simulink library "csu_esf_est_switch_frame_lib"  (R2015b)
settings: Solver=ode45  StartTime=0.0  StopTime=10.0  RelTol=1e-3
values from neighbouring files (symbols this model uses):
  esf_takeoff_accel_limit = 1.05    [csu_esf_est_switch_frame_init.m]
undefined symbols (not defined in the file or in its folder): ekf_covariance_init, kfl_accel_init, kfl_altitude_init, kfl_convergence_init, kfl_landed_init, kfl_quat_init, kfl_rate_init, kfl_state_init
libraries: simulink x2, util_info_lib x2, csu_egm_estimated_gravity_model_lib x2, util_fsw_frame_rotation_lib x2, util_common_lib x2
settings Model: Creator=escrane  LastModifiedBy=Mark Agbayani
settings DataIOCC: SaveFormat=Array
settings DebuggingCC: UnderspecifiedInitializationDetection=Classic  MergeDetectMultiDrivingBlocksExec=none  SolverPrmCheckMsg=warning  StateNameClashWarn=warning
settings HardwareCC: ProdBitPerPointer=32  ProdLargestAtomicFloat=None  ProdIntDivRoundTo=Undefined  ProdEndianess=Unspecified  ProdWordSize=32  ProdHWDeviceType=32-bit Generic
settings GRTTargetCC: GeneratePreprocessorConditionals=Disable all
settings ConfigComp: CovModelRefEnable=Off  CovSFcnEnable=off

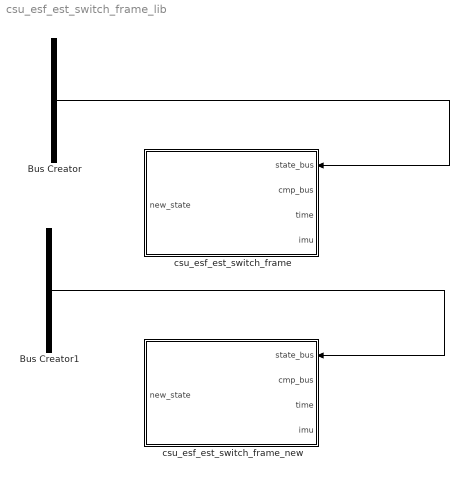
== system csu_esf_est_switch_frame_lib ==
  Bus Creator : BusCreator  Inputs=5
  Bus Creator1 : BusCreator  Inputs=6
  csu_esf_est_switch_frame : Subsystem
  csu_esf_est_switch_frame_new : Subsystem
  wires:
  Bus Creator/1 -> csu_esf_est_switch_frame/1(state_bus)
  ? -> Bus Creator/1  "x"
  ? -> Bus Creator/2  "accel"
  ? -> Bus Creator/3  "rate"
  ? -> Bus Creator/4  "q"
  ? -> Bus Creator/5  "P"
  Bus Creator1/1 -> csu_esf_est_switch_frame_new/1(state_bus)
  ? -> Bus Creator1/1  "x"
  ? -> Bus Creator1/2  "accel"
  ? -> Bus Creator1/3  "rate"
  ? -> Bus Creator1/5  "P"
  ? -> Bus Creator1/6  "altitude"
  ? -> Bus Creator1/4  "q"

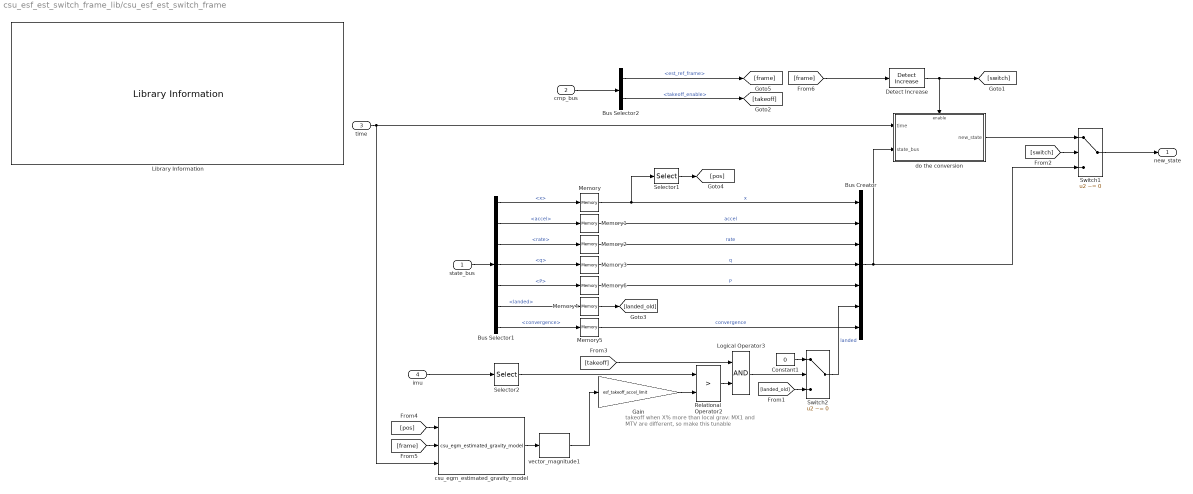
== system csu_esf_est_switch_frame_lib/csu_esf_est_switch_frame ==
  note: takeoff when X% more than local grav:
      | MX1 and MTV are different, so make this tunable
  state_bus : Inport
  cmp_bus : Inport  Port=2
  time : Inport  Port=3
  imu : Inport  Port=4
  Bus Creator : BusCreator  Inputs=7
  Bus Selector1 : BusSelector  OutputSignals=x,accel,rate,q,P,landed,convergence
  Bus Selector2 : BusSelector  OutputSignals=est_ref_frame,takeoff_enable
  Constant1 : Constant  Value=0
  Detect Increase : simulink/Logic and Bit Operations/Detect Increase  vinit=1  InputProcessing=Inherited  OutDataTypeStr=boolean
  Gain : Gain  Gain=esf_takeoff_accel_limit
  Library Information : util_info_lib/Library Information  owner='escrane'
  Logical Operator3 : Logic  AllPortsSameDT=off  OutDataTypeStr=boolean
  Memory : Memory  X0=kfl_state_init  InheritSampleTime=on
  Memory1 : Memory  X0=kfl_accel_init  InheritSampleTime=on
  Memory2 : Memory  X0=kfl_rate_init  InheritSampleTime=on
  Memory3 : Memory  X0=kfl_quat_init  InheritSampleTime=on
  Memory4 : Memory  X0=kfl_landed_init  InheritSampleTime=on
  Memory5 : Memory  X0=kfl_convergence_init  InheritSampleTime=on
  Memory6 : Memory  X0=ekf_covariance_init  InheritSampleTime=on
  Relational Operator2 : RelationalOperator  Operator=>  OutDataTypeStr=boolean
  Selector1 : Selector  InputPortWidth=kfl_n_state  IndexOptions=Index vector (dialog)  Indices=kfl_pos_index  OutputSizes=1
  Selector2 : Selector  NumberOfDimensions=2  InputPortWidth=3  IndexOptions=Index vector (dialog),Index vector (dialog)  Indices=1,3  OutputSizes=1,1
  Switch1 : Switch  Criteria=u2 ~= 0  Threshold=0.5  InputSameDT=on
  Switch2 : Switch  Criteria=u2 ~= 0  Threshold=0.5  InputSameDT=on
  csu_egm_estimated_gravity_model : csu_egm_estimated_gravity_model_lib/csu_egm_estimated_gravity_model
  do the conversion : Subsystem
  vector_magnitude1 : util_common_lib/vector_magnitude  SystemSampleTime=-1
  new_state : Outport
  wires:
  Gain/1 -> Relational Operator2/2
  csu_egm_estimated_gravity_model/1 -> vector_magnitude1/1
  [frame] -> Detect Increase/1
  [frame] -> csu_egm_estimated_gravity_model/2
  [pos] -> csu_egm_estimated_gravity_model/1
  Selector1/1 -> [pos]
  Memory5/1 -> Bus Creator/7  "convergence"
  Bus Selector1/7 -> Memory5/1  "<convergence>"
  [landed_old] -> Switch2/3
  Memory4/1 -> [landed_old]
  Bus Selector2/2 -> [takeoff]  "<takeoff_enable>"
  imu/1 -> Selector2/1
  Constant1/1 -> Switch2/1
  Switch2/1 -> Bus Creator/6  "landed"
  Logical Operator3/1 -> Switch2/2
  [takeoff] -> Logical Operator3/1
  Selector2/1 -> Relational Operator2/1
  Relational Operator2/1 -> Logical Operator3/2
  vector_magnitude1/1 -> Gain/1
  Bus Selector1/6 -> Memory4/1  "<landed>"
  state_bus/1 -> Bus Selector1/1
  Memory/1 -> Bus Creator/1, Selector1/1  "x"
  Memory1/1 -> Bus Creator/2  "accel"
  Memory2/1 -> Bus Creator/3  "rate"
  Memory3/1 -> Bus Creator/4  "q"
  Memory6/1 -> Bus Creator/5  "P"
  Bus Selector2/1 -> [frame]  "<est_ref_frame>"
  Detect Increase/1 -> [switch], do the conversion/Enable
  do the conversion/1(new_state) -> Switch1/1
  [switch] -> Switch1/2
  Bus Selector1/1 -> Memory/1  "<x>"
  Bus Selector1/2 -> Memory1/1  "<accel>"
  Bus Selector1/3 -> Memory2/1  "<rate>"
  Bus Selector1/4 -> Memory3/1  "<q>"
  Bus Selector1/5 -> Memory6/1  "<P>"
  Bus Creator/1 -> Switch1/3, do the conversion/2(state_bus)
  cmp_bus/1 -> Bus Selector2/1
  time/1 -> csu_egm_estimated_gravity_model/3, do the conversion/1(time)
  Switch1/1 -> new_state/1

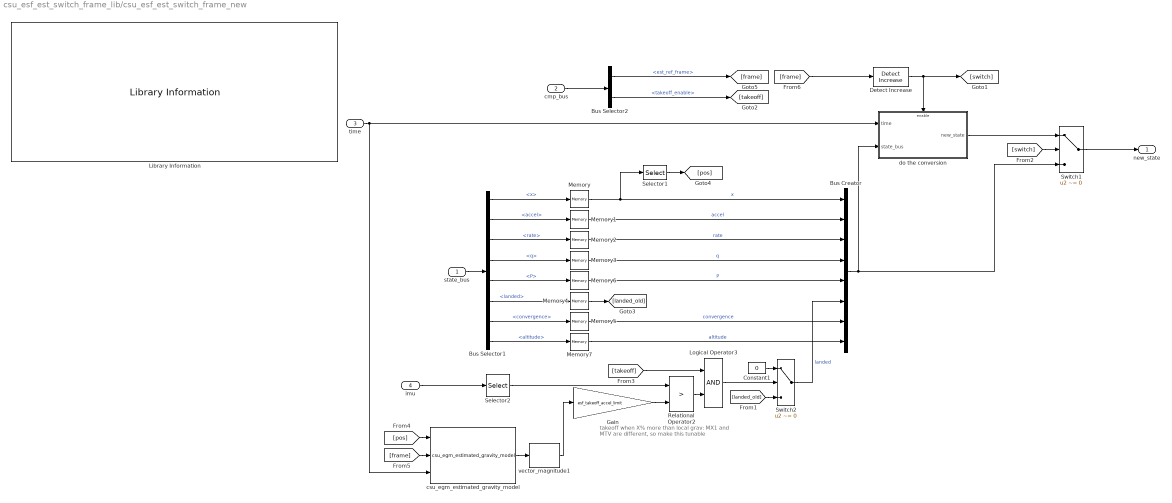
== system csu_esf_est_switch_frame_lib/csu_esf_est_switch_frame_new ==
  note: takeoff when X% more than local grav:
      | MX1 and MTV are different, so make this tunable
  state_bus : Inport
  cmp_bus : Inport  Port=2
  time : Inport  Port=3
  imu : Inport  Port=4
  Bus Creator : BusCreator  Inputs=8
  Bus Selector1 : BusSelector  OutputSignals=x,accel,rate,q,P,landed,convergence,altitude
  Bus Selector2 : BusSelector  OutputSignals=est_ref_frame,takeoff_enable
  Constant1 : Constant  Value=0
  Detect Increase : simulink/Logic and Bit Operations/Detect Increase  vinit=1  InputProcessing=Inherited  OutDataTypeStr=boolean
  Gain : Gain  Gain=esf_takeoff_accel_limit
  Library Information : util_info_lib/Library Information  owner='escrane'
  Logical Operator3 : Logic  AllPortsSameDT=off  OutDataTypeStr=boolean
  Memory : Memory  X0=kfl_state_init  InheritSampleTime=on
  Memory1 : Memory  X0=kfl_accel_init  InheritSampleTime=on
  Memory2 : Memory  X0=kfl_rate_init  InheritSampleTime=on
  Memory3 : Memory  X0=kfl_quat_init  InheritSampleTime=on
  Memory4 : Memory  X0=kfl_landed_init  InheritSampleTime=on
  Memory5 : Memory  X0=kfl_convergence_init  InheritSampleTime=on
  Memory6 : Memory  X0=ekf_covariance_init  InheritSampleTime=on
  Memory7 : Memory  X0=kfl_altitude_init  InheritSampleTime=on
  Relational Operator2 : RelationalOperator  Operator=>  OutDataTypeStr=boolean
  Selector1 : Selector  InputPortWidth=kfl_n_state  IndexOptions=Index vector (dialog)  Indices=kfl_pos_index  OutputSizes=1
  Selector2 : Selector  NumberOfDimensions=2  InputPortWidth=3  IndexOptions=Index vector (dialog),Index vector (dialog)  Indices=1,3  OutputSizes=1,1
  Switch1 : Switch  Criteria=u2 ~= 0  Threshold=0.5  InputSameDT=on
  Switch2 : Switch  Criteria=u2 ~= 0  Threshold=0.5  InputSameDT=on
  csu_egm_estimated_gravity_model : csu_egm_estimated_gravity_model_lib/csu_egm_estimated_gravity_model
  do the conversion : Subsystem
  vector_magnitude1 : util_common_lib/vector_magnitude  SystemSampleTime=-1
  new_state : Outport
  wires:
  Memory7/1 -> Bus Creator/8  "altitude"
  Bus Selector1/8 -> Memory7/1  "<altitude>"
  Gain/1 -> Relational Operator2/2
  csu_egm_estimated_gravity_model/1 -> vector_magnitude1/1
  [frame] -> Detect Increase/1
  [frame] -> csu_egm_estimated_gravity_model/2
  [pos] -> csu_egm_estimated_gravity_model/1
  Selector1/1 -> [pos]
  Memory5/1 -> Bus Creator/7  "convergence"
  Bus Selector1/7 -> Memory5/1  "<convergence>"
  [landed_old] -> Switch2/3
  Memory4/1 -> [landed_old]
  Bus Selector2/2 -> [takeoff]  "<takeoff_enable>"
  imu/1 -> Selector2/1
  Constant1/1 -> Switch2/1
  Switch2/1 -> Bus Creator/6  "landed"
  Logical Operator3/1 -> Switch2/2
  [takeoff] -> Logical Operator3/1
  Selector2/1 -> Relational Operator2/1
  Relational Operator2/1 -> Logical Operator3/2
  vector_magnitude1/1 -> Gain/1
  Bus Selector1/6 -> Memory4/1  "<landed>"
  state_bus/1 -> Bus Selector1/1
  Memory/1 -> Bus Creator/1, Selector1/1  "x"
  Memory1/1 -> Bus Creator/2  "accel"
  Memory2/1 -> Bus Creator/3  "rate"
  Memory3/1 -> Bus Creator/4  "q"
  Memory6/1 -> Bus Creator/5  "P"
  Bus Selector2/1 -> [frame]  "<est_ref_frame>"
  Detect Increase/1 -> [switch], do the conversion/Enable
  do the conversion/1(new_state) -> Switch1/1
  [switch] -> Switch1/2
  Bus Selector1/1 -> Memory/1  "<x>"
  Bus Selector1/2 -> Memory1/1  "<accel>"
  Bus Selector1/3 -> Memory2/1  "<rate>"
  Bus Selector1/4 -> Memory3/1  "<q>"
  Bus Selector1/5 -> Memory6/1  "<P>"
  Bus Creator/1 -> Switch1/3, do the conversion/2(state_bus)
  cmp_bus/1 -> Bus Selector2/1
  time/1 -> csu_egm_estimated_gravity_model/3, do the conversion/1(time)
  Switch1/1 -> new_state/1

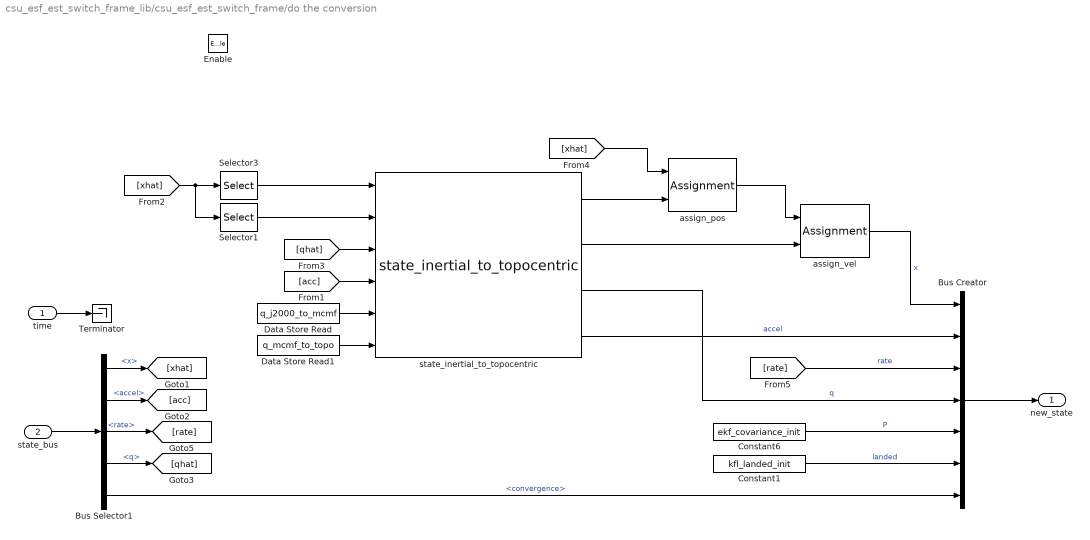
== system csu_esf_est_switch_frame_lib/csu_esf_est_switch_frame/do the conversion ==
  time : Inport
  state_bus : Inport  Port=2
  Enable : EnablePort
  Bus Creator : BusCreator  Inputs=7
  Bus Selector1 : BusSelector  OutputSignals=x,accel,rate,q,convergence
  Constant1 : Constant  Value=kfl_landed_init
  Constant6 : Constant  Value=ekf_covariance_init
  Data Store Read : DataStoreRead  DataStoreName=q_j2000_to_mcmf
  Data Store Read1 : DataStoreRead  DataStoreName=q_mcmf_to_topo
  Selector1 : Selector  InputPortWidth=kfl_n_state  IndexOptions=Index vector (dialog)  Indices=kfl_vel_index  OutputSizes=1
  Selector3 : Selector  InputPortWidth=kfl_n_state  IndexOptions=Index vector (dialog)  Indices=kfl_pos_index  OutputSizes=1
  Terminator : Terminator
  assign_pos : Assignment  IndexOptions=Index vector (dialog)  Indices=kfl_pos_index  OutputSizes=1
  assign_vel : Assignment  IndexOptions=Index vector (dialog)  Indices=kfl_vel_index  OutputSizes=1
  state_inertial_to_topocentric : util_fsw_frame_rotation_lib/state_inertial_to_topocentric  SystemSampleTime=-1
  new_state : Outport
  wires:
  time/1 -> Terminator/1
  Data Store Read/1 -> state_inertial_to_topocentric/5
  Data Store Read1/1 -> state_inertial_to_topocentric/6
  Bus Selector1/5 -> Bus Creator/7  "<convergence>"
  Constant1/1 -> Bus Creator/6  "landed"
  state_bus/1 -> Bus Selector1/1
  Bus Selector1/1 -> [xhat]  "<x>"
  Bus Selector1/2 -> [acc]  "<accel>"
  Bus Selector1/3 -> [rate]  "<rate>"
  Bus Selector1/4 -> [qhat]  "<q>"
  Bus Creator/1 -> new_state/1
  [rate] -> Bus Creator/3  "rate"
  [acc] -> state_inertial_to_topocentric/4
  [qhat] -> state_inertial_to_topocentric/3
  Constant6/1 -> Bus Creator/5  "P"
  state_inertial_to_topocentric/4 -> Bus Creator/2  "accel"
  state_inertial_to_topocentric/3 -> Bus Creator/4  "q"
  [xhat] -> Selector1/1, Selector3/1
  Selector3/1 -> state_inertial_to_topocentric/1
  Selector1/1 -> state_inertial_to_topocentric/2
  [xhat] -> assign_pos/1
  state_inertial_to_topocentric/1 -> assign_pos/2
  state_inertial_to_topocentric/2 -> assign_vel/2
  assign_pos/1 -> assign_vel/1
  assign_vel/1 -> Bus Creator/1  "x"

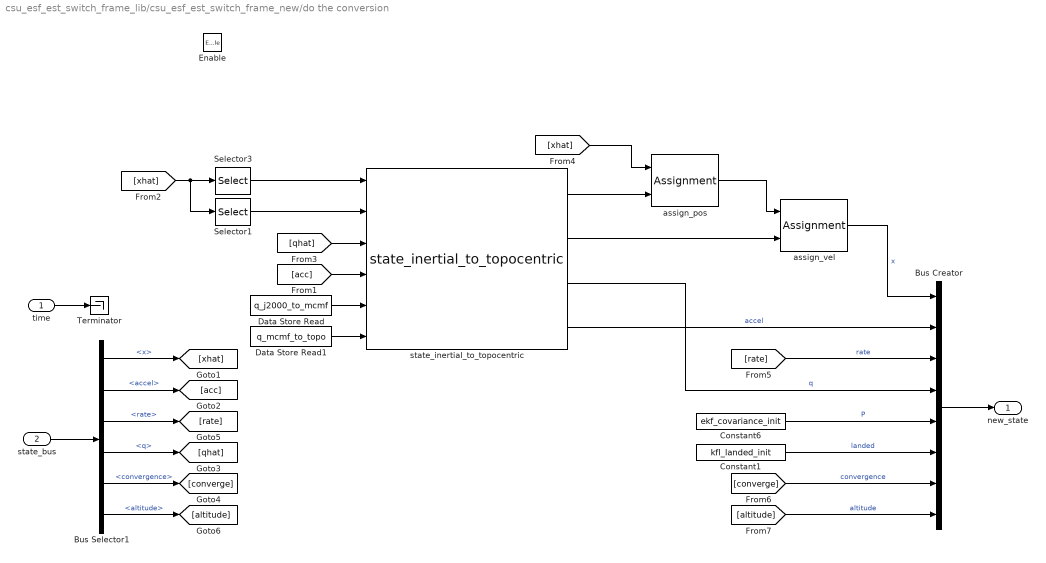
== system csu_esf_est_switch_frame_lib/csu_esf_est_switch_frame_new/do the conversion ==
  time : Inport
  state_bus : Inport  Port=2
  Enable : EnablePort
  Bus Creator : BusCreator  Inputs=8
  Bus Selector1 : BusSelector  OutputSignals=x,accel,rate,q,convergence,altitude
  Constant1 : Constant  Value=kfl_landed_init
  Constant6 : Constant  Value=ekf_covariance_init
  Data Store Read : DataStoreRead  DataStoreName=q_j2000_to_mcmf
  Data Store Read1 : DataStoreRead  DataStoreName=q_mcmf_to_topo
  Selector1 : Selector  InputPortWidth=kfl_n_state  IndexOptions=Index vector (dialog)  Indices=kfl_vel_index  OutputSizes=1
  Selector3 : Selector  InputPortWidth=kfl_n_state  IndexOptions=Index vector (dialog)  Indices=kfl_pos_index  OutputSizes=1
  Terminator : Terminator
  assign_pos : Assignment  IndexOptions=Index vector (dialog)  Indices=kfl_pos_index  OutputSizes=1
  assign_vel : Assignment  IndexOptions=Index vector (dialog)  Indices=kfl_vel_index  OutputSizes=1
  state_inertial_to_topocentric : util_fsw_frame_rotation_lib/state_inertial_to_topocentric  SystemSampleTime=-1
  new_state : Outport
  wires:
  [converge] -> Bus Creator/7  "convergence"
  [altitude] -> Bus Creator/8  "altitude"
  Bus Selector1/6 -> [altitude]  "<altitude>"
  Bus Selector1/5 -> [converge]  "<convergence>"
  time/1 -> Terminator/1
  Data Store Read/1 -> state_inertial_to_topocentric/5
  Data Store Read1/1 -> state_inertial_to_topocentric/6
  Constant1/1 -> Bus Creator/6  "landed"
  state_bus/1 -> Bus Selector1/1
  Bus Selector1/1 -> [xhat]  "<x>"
  Bus Selector1/2 -> [acc]  "<accel>"
  Bus Selector1/3 -> [rate]  "<rate>"
  Bus Selector1/4 -> [qhat]  "<q>"
  Bus Creator/1 -> new_state/1
  [rate] -> Bus Creator/3  "rate"
  [acc] -> state_inertial_to_topocentric/4
  [qhat] -> state_inertial_to_topocentric/3
  Constant6/1 -> Bus Creator/5  "P"
  state_inertial_to_topocentric/4 -> Bus Creator/2  "accel"
  state_inertial_to_topocentric/3 -> Bus Creator/4  "q"
  [xhat] -> Selector1/1, Selector3/1
  Selector3/1 -> state_inertial_to_topocentric/1
  Selector1/1 -> state_inertial_to_topocentric/2
  [xhat] -> assign_pos/1
  state_inertial_to_topocentric/1 -> assign_pos/2
  state_inertial_to_topocentric/2 -> assign_vel/2
  assign_pos/1 -> assign_vel/1
  assign_vel/1 -> Bus Creator/1  "x"
